simulink model "c_citation"  (R2020a)
settings: Solver=ode5  StartTime=0.0  StopTime=inf  FixedStep=0.01  RelTol=1e-3
InitFcn:
  | load('simulation_parameters');
values from neighbouring files (symbols this model uses):
  chord = 1.991    [citdata.mat]
  cv1 = 20000    [gear_params.m]
  cv2 = cv1    (= 20000)    [gear_params.m]
  cv3 = 4000    [gear_params.m]
  cv4 = 20000    [gear_params.m]
  deltagmax1 = 0.25    [gear_params.m]
  deltagmax2 = deltagmax1    (= 0.25)    [gear_params.m]
  deltagmax3 = 0.24    [gear_params.m]
  deltagmax4 = 0.02    [gear_params.m]
  ealphag = [0  0.2618  0.6981; 1  1.3  0.8]    [citdata.mat]
  ealphas = [0  0.2618  0.6981; 0.157  0.157  0.175]    [citdata.mat]
  g0 = 9.80665    [ac_genrl.mat]
  hDME = 0    [ac_genrl.mat]
  hGS = 0    [ac_genrl.mat]
  kt1 = 525020    [gear_params.m]
  kt2 = kt1    (= 525020)    [gear_params.m]
  kt3 = 457050    [gear_params.m]
  lh = 5.53    [citdata.mat]
  matbuaf = [0  -0.1745  0.4363; 0  -0.1  -0.1; 0.6981  -0.1  -0.1]    [citdata.mat]
  matdaf = [0 0 0.2618 0.6981 0.734842105263 0.771584210526 0.808326315789 0.845068421053 0.881810526316 0.918552631579 0.955294736842 0.992036842105 ... (529 elements, 23x23)]    [citdata.mat]
  matdam = [0 0.05 0.15 0.25 0.35 0.45 0.55 0.65 0.75 0.803571428571 0.857142857143 0.910714285714 ... (529 elements, 23x23)]    [citdata.mat]
  matdbbf = [0 0 0.6981 0.74464 0.79118 0.83772 0.88426 0.9308 0.97734 1.02388 1.07042 1.11696 ... (324 elements, 18x18)]    [citdata.mat]
  matdeaf = [0 0 0.2618 0.6981 0.734842105263 0.771584210526 0.808326315789 0.845068421053 0.881810526316 0.918552631579 0.955294736842 0.992036842105 ... (529 elements, 23x23)]    [citdata.mat]
  matdgaf = [0 0 0.2618 0.6981 -0.1745 -0.0175 -0.008 -0.009 0.4363 -0.0175 -0.008 -0.009 ... (16 elements, 4x4)]    [citdata.mat]
  matdqaf = [0 0 0.2618 0.6981 0.734842105263 0.771584210526 0.808326315789 0.845068421053 0.881810526316 0.918552631579 0.955294736842 0.992036842105 ... (529 elements, 23x23)]    [citdata.mat]
  matduaf = [0 0 0.2618 0.6981 0.734842105263 0.771584210526 0.808326315789 0.845068421053 0.881810526316 0.918552631579 0.955294736842 0.992036842105 ... (529 elements, 23x23)]    [citdata.mat]
  matdwaw = [0 0 0.1745 0.3491 0.5236 0.6458 1.2916 -0.1745 0 0.0018 0.0046 0.0088 ... (49 elements, 7x7)]    [citdata.mat]
  matedhr = [0 1 1 0.71 2 0.51 3 0.34 5 0.12 7.5 0.03 ... (20 elements, 2x10)]    [citdata.mat]
  mateif = [0  0.2618  0.6981; 0  -0.075  -0.075]    [citdata.mat]
  matelhr = [0 1 1 0.95 2 0.91 3 0.84 5 0.71 7.5 0.35 ... (20 elements, 2x10)]    [citdata.mat]
  matemhr = [0 1 1 0.9 2 0.8 3 0.7 5 0.5 7.5 0.25 ... (20 elements, 2x10)]    [citdata.mat]
  matemv1 = [0  90  100; 0  1  1]    [citdata.mat]
  matemv2 = [20  75  90; 0  1  1]    [citdata.mat]
  matemve = [0  90  100; 0  1  1]    [citdata.mat]
  matetam = [0  -0.1745  0.4363; 0  -0.04  -0.04; 1  -0.04  -0.04]    [citdata.mat]
  mateuaf = [0 0 0.6981 0.733005 0.76791 0.802815 0.83772 0.872625 0.90753 0.942435 0.97734 1.012245 ... (529 elements, 23x23)]    [citdata.mat]
  matfaaf = [0 0 0.2618 0.6981 0.734842105263 0.771584210526 0.808326315789 0.845068421053 0.881810526316 0.918552631579 0.955294736842 0.992036842105 ... (529 elements, 23x23)]    [citdata.mat]
  matfaxl = [0.15  0.35; 1  1]    [citdata.mat]
  matibaf = [0 0 0.2618 0.6981 -0.2 -0.119 -0.117 -0.108 0.3 -0.059 -0.052 -0.038 ... (16 elements, 4x4)]    [citdata.mat]
  matibb = [0 0 0.2618 1.571 3.142 -0.2 0 0 0.074 0.124 0 0 ... (50 elements, 5x10)]    [citdata.mat]
  matibmh = [0 0 15000 17142.8571429 19285.7142857 21428.5714286 23571.4285714 25714.2857143 27857.1428571 30000 0 0 ... (100 elements, 10x10)]    [citdata.mat]
  matipaf = [0  -0.1745  0.4363; 0  -0.44  -0.44; 0.6981  -0.44  -0.44]    [citdata.mat]
  matipmh = [0 0 15000 17142.8571429 19285.7142857 21428.5714286 23571.4285714 25714.2857143 27857.1428571 30000 0 0 ... (100 elements, 10x10)]    [citdata.mat]
  matiraf = [0 0 0.2618 0.6981 -0.2 0.05 -0.03 0.01 0.3 0.3 0.37 0.41 ... (16 elements, 4x4)]    [citdata.mat]
  matiuaf = [0  -0.2  0.3; 0  0.052  -0.003; 0.6981  0.052  -0.003]    [citdata.mat]
  matiwaf = [0  -0.1745  0.4363; 0  -0.185  -0.185; 0.6981  -0.185  -0.185]    [citdata.mat]
  matlaf = [0 0 0.2618 0.6981 0.734842105263 0.771584210526 0.808326315789 0.845068421053 0.881810526316 0.918552631579 0.955294736842 0.992036842105 ... (529 elements, 23x23)]    [citdata.mat]
  matlam = [0 0.05 0.15 0.25 0.35 0.45 0.55 0.65 0.75 0.803571428571 0.857142857143 0.910714285714 ... (529 elements, 23x23)]    [citdata.mat]
  matleaf = [0 0 0.2618 0.6981 0.734842105263 0.771584210526 0.808326315789 0.845068421053 0.881810526316 0.918552631579 0.955294736842 0.992036842105 ... (529 elements, 23x23)]    [citdata.mat]
  matleam = [0  -0.1745  0.4363; 0  0.58  0.58; 1  0.58  0.58]    [citdata.mat]
  matlgaf = [0 0 0.2618 0.6981 -0.1745 0.045 0.105 0.14 0.4363 0.045 0.105 0.14 ... (16 elements, 4x4)]    [citdata.mat]
  matlqaf = [0 0 0.2618 0.6981 0.734842105263 0.771584210526 0.808326315789 0.845068421053 0.881810526316 0.918552631579 0.955294736842 0.992036842105 ... (529 elements, 23x23)]    [citdata.mat]
  matluaf = [0 0 0.2618 0.6981 0.734842105263 0.771584210526 0.808326315789 0.845068421053 0.881810526316 0.918552631579 0.955294736842 0.992036842105 ... (529 elements, 23x23)]    [citdata.mat]
  matmaaf = [0 0 0.2618 0.6981 0.734842105263 0.771584210526 0.808326315789 0.845068421053 0.881810526316 0.918552631579 0.955294736842 0.992036842105 ... (484 elements, 22x22)]    [citdata.mat]
  matmaam = [0 0.05 0.15 0.25 0.35 0.45 0.55 0.65 0.75 0.803571428571 0.857142857143 0.910714285714 ... (484 elements, 22x22)]    [citdata.mat]
  matmaf = [0 0 0.2618 0.6981 0.734842105263 0.771584210526 0.808326315789 0.845068421053 0.881810526316 0.918552631579 0.955294736842 0.992036842105 ... (529 elements, 23x23)]    [citdata.mat]
  matmam = [0 0.05 0.15 0.25 0.35 0.45 0.55 0.65 0.75 0.803571428571 0.857142857143 0.910714285714 ... (529 elements, 23x23)]    [citdata.mat]
  matmbbf = [0 0 0.6981 0.74464 0.79118 0.83772 0.88426 0.9308 0.97734 1.02388 1.07042 1.11696 ... (324 elements, 18x18)]    [citdata.mat]
  matmeaf = [0 0 0.2618 0.6981 0.734842105263 0.771584210526 0.808326315789 0.845068421053 0.881810526316 0.918552631579 0.955294736842 0.992036842105 ... (529 elements, 23x23)]    [citdata.mat]
  matmeam = [0 0 1 1.05 1.1 1.15 1.2 1.25 1.3 1.35 1.4 1.45 ... (529 elements, 23x23)]    [citdata.mat]
  matmgaf = [0 0 0.2618 0.6981 -0.1745 -0.01 -0.024 -0.035 0.4363 -0.01 -0.024 -0.035 ... (16 elements, 4x4)]    [citdata.mat]
  matmqaf = [0 0 0.2618 0.6981 0.734842105263 0.771584210526 0.808326315789 0.845068421053 0.881810526316 0.918552631579 0.955294736842 0.992036842105 ... (529 elements, 23x23)]    [citdata.mat]
  matmrbr = [0  0  0.5236; 0  0  0; 0.384  0.001  0.001]    [citdata.mat]
  matnbab = [0 0 0.2618 1.571 3.142 -0.2 0 0 -0.0199 -0.1049 0 0 ... (25 elements, 5x5)]    [citdata.mat]
  matnbaf = [0  -0.2  0.3; 0  0.105  0.18; 0.6981  0.105  0.18]    [citdata.mat]
  matnbmh = [0 0 15000 17142.8571429 19285.7142857 21428.5714286 23571.4285714 25714.2857143 27857.1428571 30000 0 0 ... (100 elements, 10x10)]    [citdata.mat]
  matnpaf = [0 0 0.2618 0.6981 -0.2 0.03 0.03 0.05 0.3 -0.12 -0.12 -0.2 ... (16 elements, 4x4)]    [citdata.mat]
  matnpmh = [0 0 15000 17142.8571429 19285.7142857 21428.5714286 23571.4285714 25714.2857143 27857.1428571 30000 0 0 ... (100 elements, 10x10)]    [citdata.mat]
  matnraf = [0  -0.1745  0.4363; 0  -0.21  -0.21; 0.6981  -0.21  -0.21]    [citdata.mat]
  matnuaf = [0  -0.1745  0.4363; 0  -0.101  -0.101; 0.6981  -0.101  -0.101]    [citdata.mat]
  matnwaf = [0 0 0.2618 0.6981 -0.2 -0.02 -0.037 -0.049 0.3 0.03 0.043 0.036 ... (16 elements, 4x4)]    [citdata.mat]
  matnwmh = [0 0 15000 17142.8571429 19285.7142857 21428.5714286 23571.4285714 25714.2857143 27857.1428571 30000 0 0 ... (100 elements, 10x10)]    [citdata.mat]
  matqlaf = [0  -0.1745  0.4363; 0  -1  -1; 0.6981  -1  -1]    [citdata.mat]
  matquaf = [0 0 0.6981 0.733005 0.76791 0.802815 0.83772 0.872625 0.90753 0.942435 0.97734 1.012245 ... (529 elements, 23x23)]    [citdata.mat]
  matqxl = [0.15  0.35; 1  1]    [citdata.mat]
  matqxm = [0.15  0.35; 1  1]    [citdata.mat]
  matrtam = [0  -0.1745  0.4363; 0  0.011  0.011; 1  0.011  0.011]    [citdata.mat]
  matruaf = [0  -0.1745  0.4363; 0  0.2  0.2; 0.6981  0.2  0.2]    [citdata.mat]
  matrumh = [0 0 15000 17142.8571429 19285.7142857 21428.5714286 23571.4285714 25714.2857143 27857.1428571 30000 0 0 ... (100 elements, 10x10)]    [citdata.mat]
  matuut = [0  0.5  1; 0  1.35  1]    [citdata.mat]
  matwtam = [0  -0.1745  0.4363; 0  0.011  0.011; 1  0.011  0.011]    [citdata.mat]
  matybab = [0 0 0.2618 1.571 3.142 -0.2 0 0 0.34 0.75 0 0 ... (25 elements, 5x5)]    [citdata.mat]
  matybaf = [0  -0.1745  0.4363; 0  -0.75  -0.75; 0.6981  -0.75  -0.75]    [citdata.mat]
  matyraf = [0  -0.1745  0.4363; 0  0.85  0.85; 0.6981  0.85  0.85]    [citdata.mat]
  matyuaf = [0  -0.1745  0.4363; 0  0.23  0.23; 0.6981  0.23  0.23]    [citdata.mat]
  matywaf = [0  -0.1745  0.4363; 0  -0.04  -0.04; 0.6981  -0.04  -0.04]    [citdata.mat]
  murol = 0.03*10    (= 0.3)    [gear_params.m]
  P1 = 2000    [gear_params.m]
  P2 = P1    (= 2000)    [gear_params.m]
  P3 = 2550    [gear_params.m]
  P4 = 40000    [gear_params.m]
  psiLOC = 0    [ac_genrl.mat]
  pstat0 = 101325    [ac_genrl.mat]
  S = 24.99    [citdata.mat]
  span = 13.325    [citdata.mat]
  T0 = 288.15    [ac_genrl.mat]
  tilteng = [0 0]    [citdata.mat]
  toweng = [0 0]    [citdata.mat]
  vdommyr37 = [0  0.2618  0.6981; 0  0.025  0]    [citdata.mat]
  vdommyr38 = [0  0.2618  0.6981; -0.01  0  -0.01]    [citdata.mat]
  Vw915 = 0    [initcit.m]
  winddir = 45*(pi/180)    (= 0.785398163397)    [initcit.m]
  xcgref = 6.5    [citdata.mat]
  xDME = 0    [ac_genrl.mat]
  xeng = [8.407 8.407]    [citdata.mat]
  xGS = 0    [ac_genrl.mat]
  xiacc = 3.2    [ac_genrl.mat]
  xl1 = xcg-6.858    [gear_params.m]
  xl2 = xcg-6.858    [gear_params.m]
  xl3 = xcg-2.0752    [gear_params.m]
  xl4 = xcg-12.742    [gear_params.m]
  xLOC = 0    [ac_genrl.mat]
  ycgref = 0    [citdata.mat]
  yDME = 0    [ac_genrl.mat]
  yeng = [3 -3]    [citdata.mat]
  yGS = 0    [ac_genrl.mat]
  yiacc = 0    [ac_genrl.mat]
  yl1 = 1.918    [gear_params.m]
  yl2 = -1.918    [gear_params.m]
  yl3 = 0    [gear_params.m]
  ... (+9 more)
undefined symbols (not defined in the file or in its folder): Deng, massinit, matff, matn1d, matn2d, matthr, u0, ut0, x0, xt0
(part 2 of 5)

== system c_citation/Cessna Citation 500/Citation model DASMAT/AIRCRAFT MODEL/AFM/FMaerodims ==
  Ca : Inport
  Cadot : Inport  Port=2
  Cbdot : Inport  Port=3
  x : Inport  Port=4
  yad1 : Inport  Port=5
  Prod : Product  InputSameDT=on  SaturateOnIntegerOverflow=on  OutDataTypeStr=Inherit: Same as first input
  Prod1 : Product  Inputs=3  InputSameDT=on  SaturateOnIntegerOverflow=on  OutDataTypeStr=Inherit: Same as first input
  Prod2 : Product  Inputs=3  InputSameDT=on  SaturateOnIntegerOverflow=on  OutDataTypeStr=Inherit: Same as first input
  b/V : Fcn  Expr=span/u[4]
  c/V : Fcn  Expr=chord/u[4]
  dims : Subsystem
  dims1 : Subsystem
  dims2 : Subsystem
  qdyn*S : Fcn  Expr=u[2]*S
  FMa : Outport  VectorParamsAs1DForOutWhenUnconnected=off
  FMadot : Outport  Port=2  VectorParamsAs1DForOutWhenUnconnected=off
  FMbdot : Outport  Port=3  VectorParamsAs1DForOutWhenUnconnected=off
  wires:
  Ca/1 -> Prod/1
  Prod/1 -> dims/1(FM/length)
  dims/1(FM) -> FMa/1
  yad1/1 -> qdyn*S/1
  Cbdot/1 -> Prod2/1
  qdyn*S/1 -> Prod2/2, Prod1/2, Prod/2
  Cadot/1 -> Prod1/1
  Prod1/1 -> dims1/1(F FM/length)
  dims1/1(FM) -> FMadot/1
  Prod2/1 -> dims2/1(F FM/length)
  dims2/1(FM) -> FMbdot/1
  x/1 -> b/V/1, c/V/1
  c/V/1 -> Prod1/3
  b/V/1 -> Prod2/3

== system c_citation/Cessna Citation 500/Citation model DASMAT/AIRCRAFT MODEL/AFM/FMgustdims ==
  Cag : Inport
  yad1 : Inport  Port=2
  Prod : Product  InputSameDT=on  SaturateOnIntegerOverflow=on  OutDataTypeStr=Inherit: Same as first input
  dims : Subsystem
  qdyn*S : Fcn  Expr=u[2]*S
  FMag : Outport  VectorParamsAs1DForOutWhenUnconnected=off
  wires:
  Cag/1 -> Prod/1
  Prod/1 -> dims/1(F M/length)
  yad1/1 -> qdyn*S/1
  dims/1(FM) -> FMag/1
  qdyn*S/1 -> Prod/2

== system c_citation/Cessna Citation 500/Citation model DASMAT/AIRCRAFT MODEL/AFM/Gust axes-cg transformation ==
  Cag model : Inport
  "x " : Inport  Port=2
  massinit : Inport  Port=3
  Demux1 : Demux  Outputs=[3 3 3 3]
      settings: DisplayOption=none
  Fag transformation : S-Function  FunctionName=ac_axes  Parameters=axes_CFMgust  SFunctionDeploymentMode=off  EnableBusSupport=off
  Mag transformation : S-Function  FunctionName=ac_axes  Parameters=axes_CFMgust  SFunctionDeploymentMode=off  EnableBusSupport=off
  Mux1 : Mux  Inputs=[12 3]
  Mux2 : Mux  Inputs=[12 3]
  Mux3 : Mux  Inputs=[3 3]
  Mux4 : Mux  Inputs=[12 1 1 1]
  Mux5 : Mux  Inputs=[12 12]
  Mux6 : Mux  Inputs=3
  Sum : Sum  Inputs=+-  InputSameDT=on  SaturateOnIntegerOverflow=on  OutDataTypeStr=Inherit: Same as first input
  Sum1 : Sum  InputSameDT=on  SaturateOnIntegerOverflow=on  OutDataTypeStr=Inherit: Same as first input
  Terminator_{1..5} (5 alike) : Terminator
  delta CLLbody : Fcn  Expr=(u[2]*u[6]-u[3]*u[5])/span
  delta CMbody : Fcn  Expr=(-u[1]*u[6]+u[3]*u[4])/chord
  delta CNbody : Fcn  Expr=(u[1]*u[5]-u[2]*u[4])/span
  delta Mag transformation : S-Function  FunctionName=ac_axes  Parameters=2  SFunctionDeploymentMode=off  EnableBusSupport=off
  gust : Demux  Outputs=[3 3]
      settings: DisplayOption=none
  mass cg inertia : Demux  Outputs=[1 3 4]
      settings: DisplayOption=none
  xref : Constant  Value=xcgref
  yref : Constant  Value=ycgref
  zref : Constant  Value=zcgref
  Cag : Outport  VectorParamsAs1DForOutWhenUnconnected=off
  wires:
  mass cg inertia/3 -> Terminator_5/1
  mass cg inertia/1 -> Terminator_4/1
  Demux1/4 -> Terminator_3/1
  Demux1/2 -> Terminator_2/1
  Demux1/1 -> Terminator_1/1
  Cag model/1 -> gust/1
  massinit/1 -> mass cg inertia/1
  gust/1 -> Mux1/2
  xref/1 -> Mux6/1
  yref/1 -> Mux6/2
  zref/1 -> Mux6/3
  mass cg inertia/2 -> Sum/2
  Mux6/1 -> Sum/1
  Fag transformation/1 -> Demux1/1, Mux5/1
  Mag transformation/1 -> Sum1/1
  Sum1/1 -> Mux5/2
  Mux5/1 -> Cag/1
  Mux1/1 -> Fag transformation/1
  delta Mag transformation/1 -> Sum1/2
  Mux2/1 -> Mag transformation/1
  Sum/1 -> Mux3/2
  gust/2 -> Mux2/2
  "x "/1 -> Mux2/1, Mux1/1, Mux4/1
  Mux3/1 -> delta CLLbody/1, delta CNbody/1, delta CMbody/1
  delta CLLbody/1 -> Mux4/2
  delta CMbody/1 -> Mux4/3
  delta CNbody/1 -> Mux4/4
  Demux1/3 -> Mux3/1
  Mux4/1 -> delta Mag transformation/1

== system c_citation/Cessna Citation 500/Citation model DASMAT/AIRCRAFT MODEL/EFM/Engine axes-cg transformation ==
  FMt model : Inport
  "x " : Inport  Port=2
  massinit : Inport  Port=3
  Demux : Demux  Outputs=[3 3 3 3]
      settings: DisplayOption=none
  Ft transformation : S-Function  FunctionName=ac_axes  Parameters=2  SFunctionDeploymentMode=off  EnableBusSupport=off
  Mt transformation : S-Function  FunctionName=ac_axes  Parameters=2  SFunctionDeploymentMode=off  EnableBusSupport=off
  Mux1 : Mux  Inputs=[12 3]
  Mux2 : Mux  Inputs=[12 3]
  Mux3 : Mux  Inputs=[3 3]
  Mux4 : Mux  Inputs=[12 1 1 1]
  Mux5 : Mux  Inputs=[12 12]
  "Neg " : Gain  Gain=-1  SaturateOnIntegerOverflow=on  OutDataTypeStr=Inherit: Same as input  ParamDataTypeStr=Inherit: Same as input
  Sum1 : Sum  InputSameDT=on  SaturateOnIntegerOverflow=on  OutDataTypeStr=Inherit: Same as first input
  Terminator_{1..5} (5 alike) : Terminator
  delta LLbody : Fcn  Expr=u[2]*u[6]-u[3]*u[5]
  delta Mbody : Fcn  Expr=-u[1]*u[6]+u[3]*u[4]
  delta Mt transformation : S-Function  FunctionName=ac_axes  Parameters=2  SFunctionDeploymentMode=off  EnableBusSupport=off
  delta Nbody : Fcn  Expr=u[1]*u[5]-u[2]*u[4]
  engine : Demux  Outputs=[3 3]
      settings: DisplayOption=none
  mass cg inertia : Demux  Outputs=[1 3 4]
      settings: DisplayOption=none
  FMt : Outport  VectorParamsAs1DForOutWhenUnconnected=off
  wires:
  mass cg inertia/3 -> Terminator_5/1
  mass cg inertia/1 -> Terminator_4/1
  Demux/4 -> Terminator_3/1
  Demux/2 -> Terminator_2/1
  Demux/1 -> Terminator_1/1
  FMt model/1 -> engine/1
  massinit/1 -> mass cg inertia/1
  engine/1 -> Mux1/2
  Ft transformation/1 -> Demux/1, Mux5/1
  Mt transformation/1 -> Sum1/1
  Sum1/1 -> Mux5/2
  Mux5/1 -> FMt/1
  Mux1/1 -> Ft transformation/1
  delta Mt transformation/1 -> Sum1/2
  Mux2/1 -> Mt transformation/1
  engine/2 -> Mux2/2
  "x "/1 -> Mux2/1, Mux1/1, Mux4/1
  Mux3/1 -> delta LLbody/1, delta Nbody/1, delta Mbody/1
  delta LLbody/1 -> Mux4/2
  delta Mbody/1 -> Mux4/3
  delta Nbody/1 -> Mux4/4
  Mux4/1 -> delta Mt transformation/1
  Demux/3 -> Mux3/1
  mass cg inertia/2 -> "Neg "/1
  "Neg "/1 -> Mux3/2

== system c_citation/Cessna Citation 500/Citation model DASMAT/AIRCRAFT MODEL/EFM/Engmod ==
  x : Inport
  ut : Inport  Port=2
  yatm : Inport  Port=3
  yad1 : Inport  Port=4
  yad2 : Inport  Port=5
  Citation eng_mod : Subsystem
  Mux : Mux  Inputs=[12 2 8 2 8]
  FMt : Outport  VectorParamsAs1DForOutWhenUnconnected=off
  ypp : Outport  Port=2  VectorParamsAs1DForOutWhenUnconnected=off
  wires:
  x/1 -> Mux/1
  ut/1 -> Mux/2
  yatm/1 -> Mux/3
  yad1/1 -> Mux/4
  yad2/1 -> Mux/5
  Mux/1 -> Citation eng_mod/1(In1)
  Citation eng_mod/1(Out1) -> FMt/1
  Citation eng_mod/2(ypp) -> ypp/1

== system c_citation/Cessna Citation 500/Citation model DASMAT/AIRCRAFT MODEL/EQM/CFMa correction ==
  xdot : Inport
  FMa : Inport  Port=2
  FMadot : Inport  Port=3
  FMbdot : Inport  Port=4
  Prod2 : Product  InputSameDT=on  SaturateOnIntegerOverflow=on  OutDataTypeStr=Inherit: Same as first input
  Prod3 : Product  InputSameDT=on  SaturateOnIntegerOverflow=on  OutDataTypeStr=Inherit: Same as first input
  Sum1 : Sum  Inputs=+++  InputSameDT=on  SaturateOnIntegerOverflow=on  OutDataTypeStr=Inherit: Same as first input
  Terminator_{1..10} (10 alike) : Terminator
  derivatives : Demux  Outputs=12
      settings: DisplayOption=none
  FMa corrected : Outport  VectorParamsAs1DForOutWhenUnconnected=off
  wires:
  derivatives/12 -> Terminator_10/1
  derivatives/11 -> Terminator_9/1
  derivatives/10 -> Terminator_8/1
  derivatives/9 -> Terminator_7/1
  derivatives/8 -> Terminator_6/1
  derivatives/7 -> Terminator_5/1
  derivatives/4 -> Terminator_4/1
  derivatives/3 -> Terminator_3/1
  derivatives/2 -> Terminator_2/1
  derivatives/1 -> Terminator_1/1
  xdot/1 -> derivatives/1
  Sum1/1 -> FMa corrected/1
  FMa/1 -> Sum1/1
  FMbdot/1 -> Prod3/1
  FMadot/1 -> Prod2/1
  Prod2/1 -> Sum1/2
  Prod3/1 -> Sum1/3
  derivatives/5 -> Prod2/2
  derivatives/6 -> Prod3/2

== system c_citation/Cessna Citation 500/Citation model DASMAT/AIRCRAFT MODEL/EQM/State Derivatives ==
  note: mass
  note: inertia
  x : Inport
  FMtot : Inport  Port=2
  FMadot : Inport  Port=3
  FMbdot : Inport  Port=4
  massinit : Inport  Port=5
  wind : Inport  Port=6
  Mux1 : Mux  Inputs=[12 12]
  Mux2 : Mux  Inputs=[3 3 3 3]
  Terminator_1 : Terminator
  Vabdot : Subsystem
  aero1 : Demux  Outputs=[12 12]
      settings: DisplayOption=none
  aero2 : Demux  Outputs=[12 12]
      settings: DisplayOption=none
  eulerdot : Subsystem
  hxydot : Subsystem
  mass properties : Subsystem
  pqrdot : Subsystem
  states transformation : Subsystem
  total : Demux  Outputs=[12 12]
      settings: DisplayOption=none
  xdot : Outport  VectorParamsAs1DForOutWhenUnconnected=off
  yuvw : Outport  Port=2  VectorParamsAs1DForOutWhenUnconnected=off
  FMtot corrected : Outport  Port=3  VectorParamsAs1DForOutWhenUnconnected=off
  wires:
  states transformation/3(ydl) -> Terminator_1/1
  wind/1 -> hxydot/2(wind), Vabdot/7(wind)
  total/1 -> Vabdot/3(Ftot)
  states transformation/2(yuvw) -> hxydot/1(yuvw), yuvw/1
  Mux1/1 -> FMtot corrected/1
  hxydot/1(hxydot) -> Mux2/4
  eulerdot/1(eulerdot) -> Mux2/3
  pqrdot/2(Mtot corrected) -> Mux1/2
  pqrdot/1(pqrdot) -> Mux2/1
  Vabdot/2(Ftot corrected) -> Mux1/1
  aero2/1 -> Vabdot/5(Fbdot)
  total/2 -> pqrdot/2(Mtot)
  mass properties/2(inertia) -> pqrdot/5(inertia)
  mass properties/1(mass) -> Vabdot/6(mass)
  aero1/1 -> Vabdot/4(Fadot)
  states transformation/1(ypqr) -> pqrdot/1(ypqr), Vabdot/2(ypqr)
  x/1 -> Vabdot/1(x), eulerdot/1(x), states transformation/1(x)
  aero2/2 -> pqrdot/4(Mbdot)
  aero1/2 -> pqrdot/3(Madot)
  Vabdot/1(Vabdot) -> pqrdot/6(Vabdot), Mux2/2
  FMbdot/1 -> aero2/1
  FMadot/1 -> aero1/1
  FMtot/1 -> total/1
  massinit/1 -> mass properties/1(massinit)
  Mux2/1 -> xdot/1

== system c_citation/Cessna Citation 500/Citation model DASMAT/AIRCRAFT MODEL/LANDING GEAR/Gear axes-cg transformation ==
  FMt model : Inport
  "x " : Inport  Port=2
  massinit : Inport  Port=3
  Demux : Demux  Outputs=[3 3 3 3]
      settings: DisplayOption=none
  Ft transformation : S-Function  FunctionName=ac_axes  Parameters=2  SFunctionDeploymentMode=off  EnableBusSupport=off
  Gear Forces and Moments : Demux  Outputs=[3 3]
      settings: DisplayOption=none
  Mt transformation : S-Function  FunctionName=ac_axes  Parameters=2  SFunctionDeploymentMode=off  EnableBusSupport=off
  Mux1 : Mux  Inputs=[12 3]
  Mux2 : Mux  Inputs=[12 3]
  Mux3 : Mux  Inputs=[3 3]
  Mux4 : Mux  Inputs=[12 1 1 1]
  Mux5 : Mux  Inputs=[12 12]
  "Neg " : Gain  Gain=-1  SaturateOnIntegerOverflow=on  OutDataTypeStr=Inherit: Same as input  ParamDataTypeStr=Inherit: Same as input
  Scope3 : Scope
  Scope4 : Scope
  Terminator_{1..6} (6 alike) : Terminator
  delta LLbody : Fcn  Expr=u[2]*u[6]-u[3]*u[5]
  delta Mbody : Fcn  Expr=-u[1]*u[6]+u[3]*u[4]
  delta Mt transformation : S-Function  FunctionName=ac_axes  Parameters=2  SFunctionDeploymentMode=off  EnableBusSupport=off
  delta Nbody : Fcn  Expr=u[1]*u[5]-u[2]*u[4]
  mass cg inertia : Demux  Outputs=[1 3 4]
      settings: DisplayOption=none
  FMt : Outport  VectorParamsAs1DForOutWhenUnconnected=off
  wires:
  mass cg inertia/3 -> Terminator_5/1
  mass cg inertia/1 -> Terminator_4/1
  Demux/4 -> Terminator_3/1
  Demux/2 -> Terminator_2/1
  Demux/1 -> Terminator_1/1
  FMt model/1 -> Gear Forces and Moments/1
  massinit/1 -> mass cg inertia/1
  Gear Forces and Moments/1 -> Mux1/2
  Ft transformation/1 -> Demux/1, Mux5/1
  Mux5/1 -> FMt/1
  Mux1/1 -> Ft transformation/1
  Mux2/1 -> Mt transformation/1
  Gear Forces and Moments/2 -> Mux2/2
  "x "/1 -> Mux2/1, Mux1/1, Mux4/1
  Mux3/1 -> delta LLbody/1, delta Nbody/1, delta Mbody/1
  delta LLbody/1 -> Mux4/2
  delta Mbody/1 -> Mux4/3
  delta Nbody/1 -> Mux4/4
  Mux4/1 -> delta Mt transformation/1
  Demux/3 -> Mux3/1
  mass cg inertia/2 -> "Neg "/1
  "Neg "/1 -> Mux3/2
  Mt transformation/1 -> Scope3/1, Mux5/2, Scope4/1
  delta Mt transformation/1 -> Terminator_6/1

== system c_citation/Cessna Citation 500/Citation model DASMAT/AIRCRAFT MODEL/LANDING GEAR/Landing Gear model ==
  note: NLR Model
  x : Inport
  xdot : Inport  Port=2
  terrain elevation : Inport  Port=3
  Correct for terrain elevation : Subsystem
  Left Main Gear : Subsystem
  Mux : Mux  Inputs=2
  Mux1 : Mux  Inputs=2
  Nose Gear : Subsystem
  Right Main Gear : Subsystem
  Sum : Sum  Inputs=++++  InputSameDT=on  SaturateOnIntegerOverflow=on  OutDataTypeStr=Inherit: Same as first input
  Sum1 : Sum  Inputs=++++  InputSameDT=on  SaturateOnIntegerOverflow=on  OutDataTypeStr=Inherit: Same as first input
  Tail Scraper : Subsystem
  hdot selector : Selector  IndexOptions=Index vector (dialog)  Indices=[10]  OutputSizes=1
  Forces and Moments : Outport  VectorParamsAs1DForOutWhenUnconnected=off
  wires:
  xdot/1 -> hdot selector/1
  Mux/1 -> Left Main Gear/1(Inputs), Nose Gear/1(Inputs), Right Main Gear/1(Inputs), Tail Scraper/1(Inputs)
  Mux1/1 -> Forces and Moments/1
  Correct for terrain elevation/1(x corrected) -> Mux/1
  x/1 -> Correct for terrain elevation/1(x)
  Tail Scraper/1(FX FY FZ) -> Sum/4
  Tail Scraper/2(L M N) -> Sum1/4
  Right Main Gear/1(FX FY FZ) -> Sum/3
  Nose Gear/2(L M N) -> Sum1/2
  Sum1/1 -> Mux1/2
  Sum/1 -> Mux1/1
  Left Main Gear/1(FX FY FZ) -> Sum/1
  Left Main Gear/2(L M N) -> Sum1/1
  Nose Gear/1(FX FY FZ) -> Sum/2
  Right Main Gear/2(L M N) -> Sum1/3
  terrain elevation/1 -> Correct for terrain elevation/2(terr elev)
  hdot selector/1 -> Mux/2

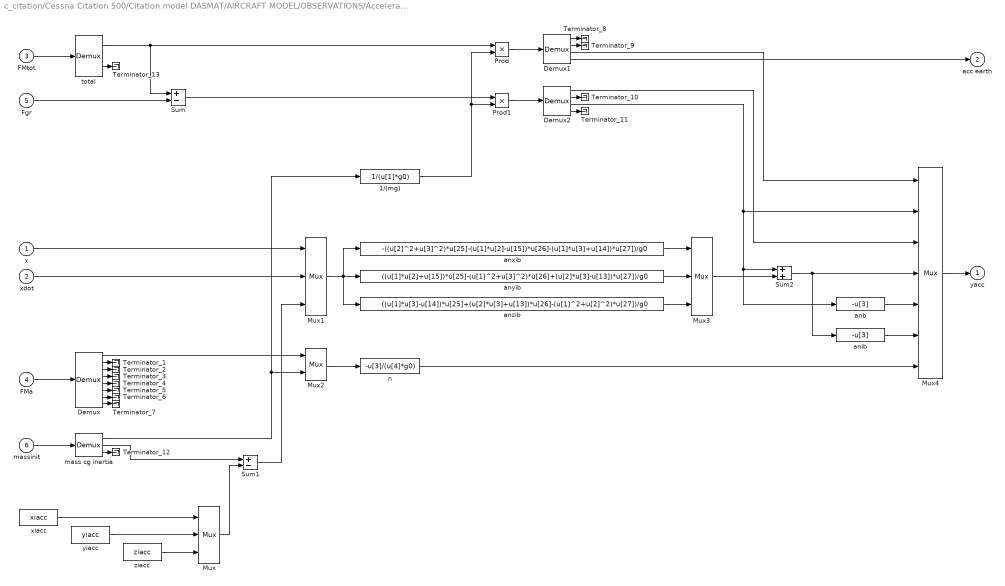
== system c_citation/Cessna Citation 500/Citation model DASMAT/AIRCRAFT MODEL/OBSERVATIONS/Acceleration ==
  x : Inport
  xdot : Inport  Port=2
  FMtot : Inport  Port=3
  FMa : Inport  Port=4
  Fgr : Inport  Port=5
  massinit : Inport  Port=6
  1/(mg) : Fcn  Expr=1/(u[1]*g0)
  Demux : Demux  Outputs=[3 3 3 3 3 3 3 3]
      settings: DisplayOption=none
  Demux1 : Demux  Outputs=[3 3 3 3]
      settings: DisplayOption=none
  Demux2 : Demux  Outputs=[3 3 3 3]
      settings: DisplayOption=none
  Mux : Mux  Inputs=3
  Mux1 : Mux  Inputs=[12 12 3]
  Mux2 : Mux  Inputs=[3 1]
  Mux3 : Mux  Inputs=3
  Mux4 : Mux  Inputs=[3 3 3 3 1 1 1]
  Prod : Product  InputSameDT=on  SaturateOnIntegerOverflow=on  OutDataTypeStr=Inherit: Same as first input
  Prod1 : Product  InputSameDT=on  SaturateOnIntegerOverflow=on  OutDataTypeStr=Inherit: Same as first input
  Sum : Sum  Inputs=+-  InputSameDT=on  SaturateOnIntegerOverflow=on  OutDataTypeStr=Inherit: Same as first input
  Sum1 : Sum  Inputs=+-  InputSameDT=on  SaturateOnIntegerOverflow=on  OutDataTypeStr=Inherit: Same as first input
  Sum2 : Sum  InputSameDT=on  SaturateOnIntegerOverflow=on  OutDataTypeStr=Inherit: Same as first input
  Terminator_{1..13} (13 alike) : Terminator
  anb : Fcn  Expr=-u[3]
  anib : Fcn  Expr=-u[3]
  anxib : Fcn  Expr=-((u[2]^2+u[3]^2)*u[25]-(u[1]*u[2]-u[15])*u[26]-(u[1]*u[3]+u[14])*u[27])/g0
  anyib : Fcn  Expr=((u[1]*u[2]+u[15])*u[25]-(u[1]^2+u[3]^2)*u[26]+(u[2]*u[3]-u[13])*u[27])/g0
  anzib : Fcn  Expr=((u[1]*u[3]-u[14])*u[25]+(u[2]*u[3]+u[13])*u[26]-(u[1]^2+u[2]^2)*u[27])/g0
  mass cg inertia : Demux  Outputs=[1 3 4]
      settings: DisplayOption=none
  n : Fcn  Expr=-u[3]/(u[4]*g0)
  total : Demux  Outputs=[12 12]
      settings: DisplayOption=none
  xiacc : Constant  Value=xiacc
  yiacc : Constant  Value=yiacc
  ziacc : Constant  Value=ziacc
  yacc : Outport  VectorParamsAs1DForOutWhenUnconnected=off
  acc earth : Outport  Port=2  VectorParamsAs1DForOutWhenUnconnected=off
  wires:
  total/2 -> Terminator_13/1
  mass cg inertia/3 -> Terminator_12/1
  Demux2/4 -> Terminator_11/1
  Demux2/2 -> Terminator_10/1
  Demux1/2 -> Terminator_9/1
  Demux1/1 -> Terminator_8/1
  Demux/8 -> Terminator_7/1
  Demux/7 -> Terminator_6/1
  Demux/6 -> Terminator_5/1
  Demux/5 -> Terminator_4/1
  Demux/4 -> Terminator_3/1
  Demux/3 -> Terminator_2/1
  Demux/2 -> Terminator_1/1
  Mux4/1 -> yacc/1
  anb/1 -> Mux4/5
  Sum1/1 -> Mux1/3
  x/1 -> Mux1/1
  xdot/1 -> Mux1/2
  mass cg inertia/2 -> Sum1/1
  anzib/1 -> Mux3/3
  anxib/1 -> Mux3/1
  anyib/1 -> Mux3/2
  Mux2/1 -> n/1
  massinit/1 -> mass cg inertia/1
  xiacc/1 -> Mux/1
  yiacc/1 -> Mux/2
  ziacc/1 -> Mux/3
  1/(mg)/1 -> Prod1/2, Prod/2
  Sum/1 -> Prod1/1
  Mux1/1 -> anxib/1, anzib/1, anyib/1
  mass cg inertia/1 -> Mux2/2, 1/(mg)/1
  Mux/1 -> Sum1/2
  Mux3/1 -> Sum2/2
  Sum2/1 -> anib/1, Mux4/4
  FMa/1 -> Demux/1
  Fgr/1 -> Sum/2
  anib/1 -> Mux4/6
  n/1 -> Mux4/7
  total/1 -> Sum/1, Prod/1
  FMtot/1 -> total/1
  Demux/1 -> Mux2/1
  Demux2/3 -> Mux4/2, Sum2/1, anb/1
  Demux1/3 -> Mux4/1
  Prod/1 -> Demux1/1
  Demux2/1 -> Mux4/3
  Prod1/1 -> Demux2/1
  Demux1/4 -> acc earth/1

== system c_citation/Cessna Citation 500/Citation model DASMAT/AIRCRAFT MODEL/OBSERVATIONS/Energy ==
  x : Inport
  xdot : Inport  Port=2
  yatm : Inport  Port=3
  Mux : Mux  Inputs=[12 12 8]
  Mux1 : Mux  Inputs=2
  spec energy : Fcn  Expr=u[10]+(u[4]*u[4])/(2*u[28])
  spec power : Fcn  Expr=u[22]+(u[4]*u[16])/u[28]
  ys : Outport  VectorParamsAs1DForOutWhenUnconnected=off
  wires:
  spec power/1 -> Mux1/2
  spec energy/1 -> Mux1/1
  x/1 -> Mux/1
  xdot/1 -> Mux/2
  Mux1/1 -> ys/1
  yatm/1 -> Mux/3
  Mux/1 -> spec power/1, spec energy/1

== system c_citation/Cessna Citation 500/Citation model DASMAT/AIRCRAFT MODEL/OBSERVATIONS/Flight-Path ==
  x : Inport
  xdot : Inport  Port=2
  yuvw : Inport  Port=3
  acc earth : Inport  Port=4
  Demux : Demux  Outputs=[3 3 3 3]
      settings: DisplayOption=none
  Mux : Mux  Inputs=[12 12 3 3]
  Mux1 : Mux  Inputs=[30 1 1]
  Mux2 : Mux  Inputs=17
  Terminator11 : Terminator
  Terminator12 : Terminator
  Terminator13 : Terminator
  Vground : Fcn  Expr=sqrt(u[23]*u[23]+u[24]*u[24]+u[22]*u[22])
  bank angle : Fcn  Expr=asin(sin(u[7])*cos(u[8]))
  chi : Fcn  Expr=atan2(u[26],u[25])
  chidot : Fcn  Expr=(u[25]*u[29]*g0-u[28]*g0*u[26])/(u[4]*u[4]-u[27]*u[27])
  chimagn : Fcn  Expr=0
  chitrue : Fcn  Expr=atan2(u[24],u[23])
  chitruedot : Fcn  Expr=(u[23]*u[29]*g0-u[28]*g0*u[24])/(u[31]*u[31]-u[22]*u[22])
  flightpath acc : Fcn  Expr=u[16]/g0
  gamma : Fcn  Expr=asin(-u[27]/u[4])
  gammadot : Fcn  Expr=(-u[4]*u[30]*g0+u[16]*u[27])/(u[4]*sqrt(u[4]*u[4]-u[27]*u[27]))
  gammatrue : Fcn  Expr=asin(u[22]/u[31])
  gammatruedot : Fcn  Expr=(u[31]*u[32]*g0-u[16]*u[22])/(u[31]*sqrt(u[31]*u[31]-u[22]*u[22]))
  gsdev : Fcn  Expr=atan2(u[10]-hGS,sqrt((xGS-u[11])*(xGS-u[11])+(yGS-u[12])*(yGS-u[12]))) - 3*pi/180
  locdev : Fcn  Expr=psiLOC - atan2(yLOC-u[12],xLOC-u[11])
  psimagn : Fcn  Expr=0
  range : Fcn  Expr=sqrt((u[11]-xDME)*(u[11]-xDME)+(u[12]-yDME)*(u[12]-yDME)+(u[10]-hDME)*(u[10]-hDME))
  vertical acc : Fcn  Expr=-u[30]
  yfp : Outport  VectorParamsAs1DForOutWhenUnconnected=off
  wires:
  Demux/3 -> Terminator13/1
  Demux/2 -> Terminator12/1
  Demux/1 -> Terminator11/1
  vertical acc/1 -> Mux1/3, Mux2/16
  Mux1/1 -> gammatruedot/1, chitruedot/1, gammatrue/1, chitrue/1
  Vground/1 -> Mux1/2, Mux2/15
  xdot/1 -> Mux/2
  Demux/4 -> Mux/3
  acc earth/1 -> Mux/4
  yuvw/1 -> Demux/1
  chi/1 -> Mux2/2
  Mux2/1 -> yfp/1
  gamma/1 -> Mux2/1
  gammadot/1 -> Mux2/3
  chidot/1 -> Mux2/4
  gammatrue/1 -> Mux2/5
  chitrue/1 -> Mux2/6
  gammatruedot/1 -> Mux2/7
  flightpath acc/1 -> Mux2/17
  range/1 -> Mux2/14
  locdev/1 -> Mux2/13
  gsdev/1 -> Mux2/12
  bank angle/1 -> Mux2/11
  psimagn/1 -> Mux2/10
  chimagn/1 -> Mux2/9
  chitruedot/1 -> Mux2/8
  x/1 -> Mux/1
  Mux/1 -> Mux1/1, gammadot/1, chi/1, gamma/1, chidot/1, gsdev/1, locdev/1, range/1, Vground/1, vertical acc/1, flightpath acc/1, bank angle/1, psimagn/1, chimagn/1

== system c_citation/Cessna Citation 500/Citation model DASMAT/AIRCRAFT MODEL/WIND//TURBULENCE/Logarithmic Wind model ==
  In1 : Inport
  He Selector : Selector  InputPortWidth=12  IndexOptions=Index vector (dialog)  Indices=[10]  OutputSizes=1
  Logarithmic Wind model : Subsystem
  Mux : Mux  Inputs=3
  Out1 : Outport  VectorParamsAs1DForOutWhenUnconnected=off
  wires:
  In1/1 -> He Selector/1
  Mux/1 -> Out1/1
  Logarithmic Wind model/1(uwind) -> Mux/1  "uwind"
  Logarithmic Wind model/2(vwind) -> Mux/2  "vwind"
  Logarithmic Wind model/3(wwind) -> Mux/3  "wwind"
  He Selector/1 -> Logarithmic Wind model/1(he)

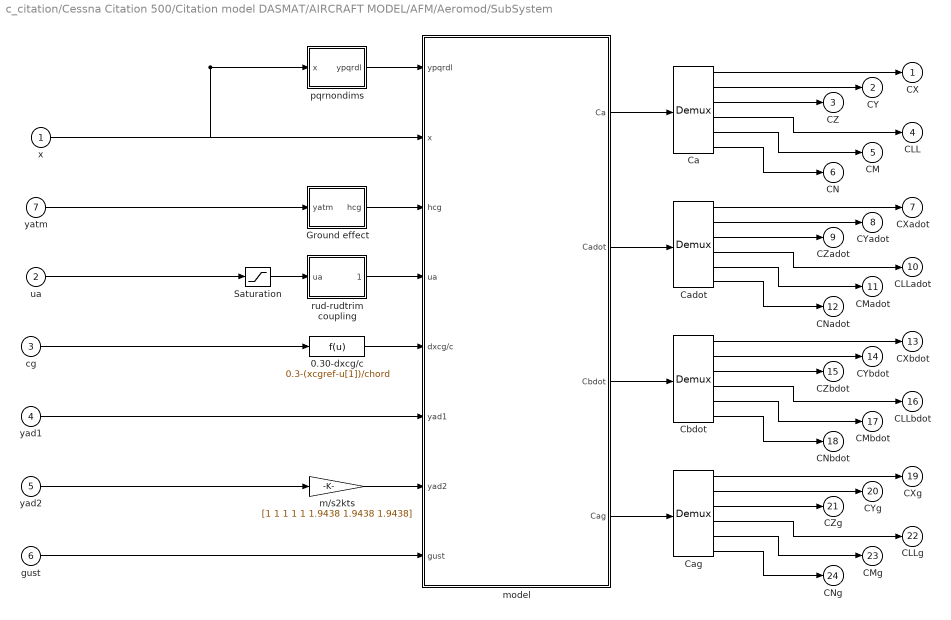
== system c_citation/Cessna Citation 500/Citation model DASMAT/AIRCRAFT MODEL/AFM/Aeromod/SubSystem ==
  x : Inport
  ua : Inport  Port=2
  cg : Inport  Port=3
  yad1 : Inport  Port=4
  yad2 : Inport  Port=5
  gust : Inport  Port=6
  yatm : Inport  Port=7
  0.30-dxcg/c : Fcn  Expr=0.3-(xcgref-u[1])/chord
  Ca : Demux  Outputs=6
      settings: DisplayOption=none
  Cadot : Demux  Outputs=6
      settings: DisplayOption=none
  Cag : Demux  Outputs=6
      settings: DisplayOption=none
  Cbdot : Demux  Outputs=6
      settings: DisplayOption=none
  Ground effect : Subsystem
  Saturation : Saturate  UpperLimit="[ 15  37  22  15  20  10 40 180/pi]*pi/180"  LowerLimit="[-20 -37 -22 -15 -20 -10 0  0]*pi/180"
  m/s2kts : Gain  Gain=[1 1 1 1 1 1.9438 1.9438 1.9438]  SaturateOnIntegerOverflow=on  OutDataTypeStr=Inherit: Same as input  ParamDataTypeStr=Inherit: Same as input
  model : Subsystem
  pqrnondims : Subsystem
  rud-rudtrim coupling : Subsystem
  CX : Outport  VectorParamsAs1DForOutWhenUnconnected=off
  CY : Outport  Port=2  VectorParamsAs1DForOutWhenUnconnected=off
  CZ : Outport  Port=3  VectorParamsAs1DForOutWhenUnconnected=off
  CLL : Outport  Port=4  VectorParamsAs1DForOutWhenUnconnected=off
  CM : Outport  Port=5  VectorParamsAs1DForOutWhenUnconnected=off
  CN : Outport  Port=6  VectorParamsAs1DForOutWhenUnconnected=off
  CXadot : Outport  Port=7  VectorParamsAs1DForOutWhenUnconnected=off
  CYadot : Outport  Port=8  VectorParamsAs1DForOutWhenUnconnected=off
  CZadot : Outport  Port=9  VectorParamsAs1DForOutWhenUnconnected=off
  CLLadot : Outport  Port=10  VectorParamsAs1DForOutWhenUnconnected=off
  CMadot : Outport  Port=11  VectorParamsAs1DForOutWhenUnconnected=off
  CNadot : Outport  Port=12  VectorParamsAs1DForOutWhenUnconnected=off
  CXbdot : Outport  Port=13  VectorParamsAs1DForOutWhenUnconnected=off
  CYbdot : Outport  Port=14  VectorParamsAs1DForOutWhenUnconnected=off
  CZbdot : Outport  Port=15  VectorParamsAs1DForOutWhenUnconnected=off
  CLLbdot : Outport  Port=16  VectorParamsAs1DForOutWhenUnconnected=off
  CMbdot : Outport  Port=17  VectorParamsAs1DForOutWhenUnconnected=off
  CNbdot : Outport  Port=18  VectorParamsAs1DForOutWhenUnconnected=off
  CXg : Outport  Port=19  VectorParamsAs1DForOutWhenUnconnected=off
  CYg : Outport  Port=20  VectorParamsAs1DForOutWhenUnconnected=off
  CZg : Outport  Port=21  VectorParamsAs1DForOutWhenUnconnected=off
  CLLg : Outport  Port=22  VectorParamsAs1DForOutWhenUnconnected=off
  CMg : Outport  Port=23  VectorParamsAs1DForOutWhenUnconnected=off
  CNg : Outport  Port=24  VectorParamsAs1DForOutWhenUnconnected=off
  wires:
  yad2/1 -> m/s2kts/1
  m/s2kts/1 -> model/7(yad2)
  Saturation/1 -> rud-rudtrim coupling/1(ua)
  model/4(Cag) -> Cag/1
  model/3(Cbdot) -> Cbdot/1
  Cbdot/2 -> CYbdot/1
  Cbdot/1 -> CXbdot/1
  Cbdot/3 -> CZbdot/1
  Cbdot/4 -> CLLbdot/1
  Cbdot/5 -> CMbdot/1
  Cbdot/6 -> CNbdot/1
  Cag/6 -> CNg/1
  Cag/5 -> CMg/1
  Cag/4 -> CLLg/1
  Cag/3 -> CZg/1
  Cag/1 -> CXg/1
  Cag/2 -> CYg/1
  model/2(Cadot) -> Cadot/1
  Cadot/2 -> CYadot/1
  Cadot/1 -> CXadot/1
  Cadot/3 -> CZadot/1
  Cadot/4 -> CLLadot/1
  Cadot/5 -> CMadot/1
  Cadot/6 -> CNadot/1
  Ca/6 -> CN/1
  Ca/5 -> CM/1
  Ca/4 -> CLL/1
  Ca/3 -> CZ/1
  Ca/1 -> CX/1
  Ca/2 -> CY/1
  model/1(Ca) -> Ca/1
  yad1/1 -> model/6(yad1)
  gust/1 -> model/8(gust)
  cg/1 -> 0.30-dxcg/c/1
  ua/1 -> Saturation/1
  x/1 -> pqrnondims/1(x), model/2(x)
  0.30-dxcg/c/1 -> model/5(dxcg/c)
  Ground effect/1(hcg) -> model/3(hcg)
  rud-rudtrim coupling/1(ua coupled) -> model/4(ua)
  pqrnondims/1(ypqrdl) -> model/1(ypqrdl)
  yatm/1 -> Ground effect/1(yatm)

== system c_citation/Cessna Citation 500/Citation model DASMAT/AIRCRAFT MODEL/AFM/FMaerodims/dims ==
  note: X,Y,Z
  FM/length : Inport
  Demux : Demux  Outputs=[12 3 3 3 3]
      settings: DisplayOption=none
  LL,M,N air : Gain  Gain=[span chord span]  SaturateOnIntegerOverflow=on  OutDataTypeStr=Inherit: Same as input  ParamDataTypeStr=Inherit: Same as input
  LL,M,N body : Gain  Gain=[span chord span]  SaturateOnIntegerOverflow=on  OutDataTypeStr=Inherit: Same as input  ParamDataTypeStr=Inherit: Same as input
  LL,M,N earth : Gain  Gain=[span chord span]  SaturateOnIntegerOverflow=on  OutDataTypeStr=Inherit: Same as input  ParamDataTypeStr=Inherit: Same as input
  LL,M,N stab : Gain  Gain=[span chord span]  SaturateOnIntegerOverflow=on  OutDataTypeStr=Inherit: Same as input  ParamDataTypeStr=Inherit: Same as input
  Mux : Mux  Inputs=[12 3 3 3 3]
  FM : Outport  VectorParamsAs1DForOutWhenUnconnected=off
  wires:
  LL,M,N earth/1 -> Mux/5
  Demux/5 -> LL,M,N earth/1
  LL,M,N body/1 -> Mux/4
  LL,M,N stab/1 -> Mux/3
  LL,M,N air/1 -> Mux/2
  Demux/1 -> Mux/1
  Demux/2 -> LL,M,N air/1
  Demux/3 -> LL,M,N stab/1
  Demux/4 -> LL,M,N body/1
  Mux/1 -> FM/1
  FM/length/1 -> Demux/1

== system c_citation/Cessna Citation 500/Citation model DASMAT/AIRCRAFT MODEL/AFM/FMaerodims/dims1 ==
  note: X,Y,Z
  F FM/length : Inport
  Demux : Demux  Outputs=[12 3 3 3 3]
      settings: DisplayOption=none
  LL,M,N air : Gain  Gain=[span chord span]  SaturateOnIntegerOverflow=on  OutDataTypeStr=Inherit: Same as input  ParamDataTypeStr=Inherit: Same as input
  LL,M,N body : Gain  Gain=[span chord span]  SaturateOnIntegerOverflow=on  OutDataTypeStr=Inherit: Same as input  ParamDataTypeStr=Inherit: Same as input
  LL,M,N earth : Gain  Gain=[span chord span]  SaturateOnIntegerOverflow=on  OutDataTypeStr=Inherit: Same as input  ParamDataTypeStr=Inherit: Same as input
  LL,M,N stab : Gain  Gain=[span chord span]  SaturateOnIntegerOverflow=on  OutDataTypeStr=Inherit: Same as input  ParamDataTypeStr=Inherit: Same as input
  Mux : Mux  Inputs=[12 3 3 3 3]
  FM : Outport  VectorParamsAs1DForOutWhenUnconnected=off
  wires:
  F FM/length/1 -> Demux/1
  Mux/1 -> FM/1
  Demux/4 -> LL,M,N body/1
  Demux/3 -> LL,M,N stab/1
  Demux/2 -> LL,M,N air/1
  Demux/1 -> Mux/1
  LL,M,N air/1 -> Mux/2
  LL,M,N stab/1 -> Mux/3
  LL,M,N body/1 -> Mux/4
  Demux/5 -> LL,M,N earth/1
  LL,M,N earth/1 -> Mux/5

== system c_citation/Cessna Citation 500/Citation model DASMAT/AIRCRAFT MODEL/AFM/FMaerodims/dims2 ==
  note: X,Y,Z
  F FM/length : Inport
  Demux : Demux  Outputs=[12 3 3 3 3]
      settings: DisplayOption=none
  LL,M,N air : Gain  Gain=[span chord span]  SaturateOnIntegerOverflow=on  OutDataTypeStr=Inherit: Same as input  ParamDataTypeStr=Inherit: Same as input
  LL,M,N body : Gain  Gain=[span chord span]  SaturateOnIntegerOverflow=on  OutDataTypeStr=Inherit: Same as input  ParamDataTypeStr=Inherit: Same as input
  LL,M,N earth : Gain  Gain=[span chord span]  SaturateOnIntegerOverflow=on  OutDataTypeStr=Inherit: Same as input  ParamDataTypeStr=Inherit: Same as input
  LL,M,N stab : Gain  Gain=[span chord span]  SaturateOnIntegerOverflow=on  OutDataTypeStr=Inherit: Same as input  ParamDataTypeStr=Inherit: Same as input
  Mux : Mux  Inputs=[12 3 3 3 3]
  FM : Outport  VectorParamsAs1DForOutWhenUnconnected=off
  wires:
  LL,M,N earth/1 -> Mux/5
  Demux/5 -> LL,M,N earth/1
  LL,M,N body/1 -> Mux/4
  LL,M,N stab/1 -> Mux/3
  LL,M,N air/1 -> Mux/2
  Demux/1 -> Mux/1
  Demux/2 -> LL,M,N air/1
  Demux/3 -> LL,M,N stab/1
  Demux/4 -> LL,M,N body/1
  Mux/1 -> FM/1
  F FM/length/1 -> Demux/1

== system c_citation/Cessna Citation 500/Citation model DASMAT/AIRCRAFT MODEL/AFM/FMgustdims/dims ==
  note: X,Y,Z
  F M/length : Inport
  Demux : Demux  Outputs=[12 3 3 3 3]
      settings: DisplayOption=none
  LL,M,N air : Gain  Gain=[span chord span]  SaturateOnIntegerOverflow=on  OutDataTypeStr=Inherit: Same as input  ParamDataTypeStr=Inherit: Same as input
  LL,M,N body : Gain  Gain=[span chord span]  SaturateOnIntegerOverflow=on  OutDataTypeStr=Inherit: Same as input  ParamDataTypeStr=Inherit: Same as input
  LL,M,N earth : Gain  Gain=[span chord span]  SaturateOnIntegerOverflow=on  OutDataTypeStr=Inherit: Same as input  ParamDataTypeStr=Inherit: Same as input
  LL,M,N stab : Gain  Gain=[span chord span]  SaturateOnIntegerOverflow=on  OutDataTypeStr=Inherit: Same as input  ParamDataTypeStr=Inherit: Same as input
  Mux : Mux  Inputs=[12 3 3 3 3]
  FM : Outport  VectorParamsAs1DForOutWhenUnconnected=off
  wires:
  LL,M,N earth/1 -> Mux/5
  Demux/5 -> LL,M,N earth/1
  LL,M,N body/1 -> Mux/4
  LL,M,N stab/1 -> Mux/3
  LL,M,N air/1 -> Mux/2
  Demux/1 -> Mux/1
  Demux/2 -> LL,M,N air/1
  Demux/3 -> LL,M,N stab/1
  Demux/4 -> LL,M,N body/1
  Mux/1 -> FM/1
  F M/length/1 -> Demux/1

== system c_citation/Cessna Citation 500/Citation model DASMAT/AIRCRAFT MODEL/EFM/Engmod/Citation eng_mod ==
  In1 : Inport
  Demux : Demux  Outputs=32
      settings: DisplayOption=none
  Mux : Mux  Inputs=6
  Mux1 : Mux  Inputs=2
  Subsystem1 : Subsystem
  Out1 : Outport  VectorParamsAs1DForOutWhenUnconnected=off
  ypp : Outport  Port=2  VectorParamsAs1DForOutWhenUnconnected=off
  wires:
  Subsystem1/4(MXt) -> Mux/4
  Subsystem1/3(Zt) -> Mux/3
  Subsystem1/2(Yt) -> Mux/2
  Subsystem1/1(Xt) -> Mux/1
  Subsystem1/6(MZt) -> Mux/6
  Subsystem1/5(MYt) -> Mux/5
  Mux/1 -> Out1/1
  In1/1 -> Demux/1
  Demux/1 -> Subsystem1/1(pbody)
  Demux/2 -> Subsystem1/2(qbody)
  Demux/3 -> Subsystem1/3(rbody)
  Demux/4 -> Subsystem1/4(VTAS)
  Demux/5 -> Subsystem1/5(alpha)
  Demux/6 -> Subsystem1/6(beta)
  Demux/7 -> Subsystem1/7(phi)
  Demux/8 -> Subsystem1/8(theta)
  Demux/9 -> Subsystem1/9(psi)
  Demux/10 -> Subsystem1/10(he)
  Demux/11 -> Subsystem1/11(xe)
  Demux/12 -> Subsystem1/12(ye)
  Demux/13 -> Subsystem1/13(ut1)
  Demux/14 -> Subsystem1/14(ut2)
  Demux/15 -> Subsystem1/15(pstat)
  Demux/16 -> Subsystem1/16(rho)
  Demux/17 -> Subsystem1/17(temp)
  Demux/18 -> Subsystem1/18(grav)
  Demux/19 -> Subsystem1/19(hpress)
  Demux/20 -> Subsystem1/20(hradio)
  Demux/21 -> Subsystem1/21(Hgeopot)
  Demux/22 -> Subsystem1/22(Vsound)
  Demux/23 -> Subsystem1/23(Mach)
  Demux/24 -> Subsystem1/24(qdyn)
  Demux/25 -> Subsystem1/25(Reynl)
  Demux/26 -> Subsystem1/26(qc)
  Demux/27 -> Subsystem1/27(qrel)
  Demux/28 -> Subsystem1/28(ptot)
  Demux/29 -> Subsystem1/29(temptot)
  Demux/30 -> Subsystem1/30(VEAS)
  Demux/31 -> Subsystem1/31(VCAS)
  Demux/32 -> Subsystem1/32(VIAS)
  Subsystem1/7(yppleft) -> Mux1/1
  Subsystem1/8(yppright) -> Mux1/2
  Mux1/1 -> ypp/1

== system c_citation/Cessna Citation 500/Citation model DASMAT/AIRCRAFT MODEL/EQM/State Derivatives/Vabdot ==
  x : Inport
  ypqr : Inport  Port=2
  Ftot : Inport  Port=3
  Fadot : Inport  Port=4
  Fbdot : Inport  Port=5
  mass : Inport  Port=6
  wind : Inport  Port=7
  Mux1 : Mux  Inputs=3
  Prod : Product  InputSameDT=on  SaturateOnIntegerOverflow=on  OutDataTypeStr=Inherit: Same as first input
  Prod1 : Product  InputSameDT=on  SaturateOnIntegerOverflow=on  OutDataTypeStr=Inherit: Same as first input
  Sum : Sum  Inputs=+++  InputSameDT=on  SaturateOnIntegerOverflow=on  OutDataTypeStr=Inherit: Same as first input
  Vdot : Subsystem
  abdot : Subsystem
  winddot : Derivative
  Vabdot : Outport  VectorParamsAs1DForOutWhenUnconnected=off
  Ftot corrected : Outport  Port=2  VectorParamsAs1DForOutWhenUnconnected=off
  wires:
  wind/1 -> winddot/1, Vdot/5(wind), abdot/7(wind)
  winddot/1 -> abdot/8(winddot), Vdot/6(winddot)
  Vdot/1(Vdot) -> Mux1/1
  mass/1 -> Vdot/4(mass), abdot/6(mass)
  ypqr/1 -> Vdot/2(ypqr), abdot/2(ypqr)
  x/1 -> Vdot/1(x), abdot/1(x)
  abdot/1(adot) -> Vdot/7(adot), Prod/2, Mux1/2
  abdot/2(bdot) -> Vdot/8(bdot), Prod1/2, Mux1/3
  Fbdot/1 -> abdot/5(Fbdot), Prod1/1
  Fadot/1 -> abdot/4(Fadot), Prod/1
  Prod1/1 -> Sum/3
  Mux1/1 -> Vabdot/1
  Sum/1 -> Vdot/3(Ftot), Ftot corrected/1
  Prod/1 -> Sum/2
  Ftot/1 -> abdot/3(Ftot), Sum/1

== system c_citation/Cessna Citation 500/Citation model DASMAT/AIRCRAFT MODEL/EQM/State Derivatives/eulerdot ==
  x : Inport
  Mux : Mux  Inputs=3
  phidot : Fcn  Expr=u[1]+tan(u[8])*(u[2]*sin(u[7])+u[3]*cos(u[7]))
  psidot : Fcn  Expr=(u[2]*sin(u[7])+u[3]*cos(u[7]))/cos(u[8])
  thetadot : Fcn  Expr=u[2]*cos(u[7])-u[3]*sin(u[7])
  eulerdot : Outport  VectorParamsAs1DForOutWhenUnconnected=off
  wires:
  x/1 -> phidot/1, psidot/1, thetadot/1
  Mux/1 -> eulerdot/1
  phidot/1 -> Mux/1
  thetadot/1 -> Mux/2
  psidot/1 -> Mux/3

== system c_citation/Cessna Citation 500/Citation model DASMAT/AIRCRAFT MODEL/EQM/State Derivatives/hxydot ==
  yuvw : Inport
  wind : Inport  Port=2
  Demux : Demux  Outputs=[3 3 3 3]
      settings: DisplayOption=none
  Demux1 : Demux  Outputs=[3 3 3 3]
      settings: DisplayOption=none
  Mux : Mux  Inputs=[3 3]
  Mux1 : Mux  Inputs=3
  Terminator_{1..6} (6 alike) : Terminator
  hedot : Fcn  Expr=-(u[3]+u[6])
  xedot : Fcn  Expr=u[1]+u[4]
  yedot : Fcn  Expr=u[2]+u[5]
  hxydot : Outport  VectorParamsAs1DForOutWhenUnconnected=off
  wires:
  Demux1/3 -> Terminator_6/1
  Demux1/2 -> Terminator_5/1
  Demux1/1 -> Terminator_4/1
  Demux/3 -> Terminator_3/1
  Demux/2 -> Terminator_2/1
  Demux/1 -> Terminator_1/1
  wind/1 -> Demux1/1
  Demux1/4 -> Mux/2
  yedot/1 -> Mux1/3
  xedot/1 -> Mux1/2
  hedot/1 -> Mux1/1  "hedot"
  Mux1/1 -> hxydot/1
  Mux/1 -> hedot/1, yedot/1, xedot/1
  yuvw/1 -> Demux/1
  Demux/4 -> Mux/1

== system c_citation/Cessna Citation 500/Citation model DASMAT/AIRCRAFT MODEL/EQM/State Derivatives/mass properties ==
  massinit : Inport
  GAMMA : Fcn  Expr=u[1]*u[3]-u[4]*u[4]
  Mux : Mux  Inputs=[4 1]
  Mux1 : Mux  Inputs=9
  Terminator_1 : Terminator
  c1 : Fcn  Expr=((u[2]-u[3])*u[3]-u[4]*u[4])/u[5]
  c2 : Fcn  Expr=(u[1]-u[2]+u[3])*u[4]/u[5]
  c3 : Fcn  Expr=u[3]/u[5]
  c4 : Fcn  Expr=u[4]/u[5]
  c5 : Fcn  Expr=(u[3]-u[1])/u[2]
  c6 : Fcn  Expr=u[4]/u[2]
  c7 : Fcn  Expr=1/u[2]
  c8 : Fcn  Expr=((u[1]-u[2])*u[1]+u[4]*u[4])/u[5]
  c9 : Fcn  Expr=u[1]/u[5]
  mass cg inertia : Demux  Outputs=[1 3 4]
      settings: DisplayOption=none
  mass : Outport  VectorParamsAs1DForOutWhenUnconnected=off
  inertia : Outport  Port=2  VectorParamsAs1DForOutWhenUnconnected=off
  wires:
  mass cg inertia/2 -> Terminator_1/1
  massinit/1 -> mass cg inertia/1
  mass cg inertia/1 -> mass/1
  mass cg inertia/3 -> GAMMA/1, Mux/1
  GAMMA/1 -> Mux/2
  c1/1 -> Mux1/1
  c2/1 -> Mux1/2
  c3/1 -> Mux1/3
  c4/1 -> Mux1/4
  c5/1 -> Mux1/5
  c6/1 -> Mux1/6
  c7/1 -> Mux1/7
  c8/1 -> Mux1/8
  c9/1 -> Mux1/9
  Mux1/1 -> inertia/1
  Mux/1 -> c2/1, c3/1, c4/1, c5/1, c6/1, c7/1, c8/1, c9/1, c1/1

== system c_citation/Cessna Citation 500/Citation model DASMAT/AIRCRAFT MODEL/EQM/State Derivatives/pqrdot ==
  ypqr : Inport
  Mtot : Inport  Port=2
  Madot : Inport  Port=3
  Mbdot : Inport  Port=4
  inertia : Inport  Port=5
  Vabdot : Inport  Port=6
  Demux : Demux  Outputs=3
      settings: DisplayOption=none
  Demux1 : Demux  Outputs=[3 3 3 3]
      settings: DisplayOption=none
  Demux2 : Demux  Outputs=[3 3 3 3]
      settings: DisplayOption=none
  Mux : Mux  Inputs=[3 3 9]
  Mux1 : Mux  Inputs=3
  Prod : Product  InputSameDT=on  SaturateOnIntegerOverflow=on  OutDataTypeStr=Inherit: Same as first input
  Prod1 : Product  InputSameDT=on  SaturateOnIntegerOverflow=on  OutDataTypeStr=Inherit: Same as first input
  Sum : Sum  Inputs=+++  InputSameDT=on  SaturateOnIntegerOverflow=on  OutDataTypeStr=Inherit: Same as first input
  Terminator_{1..7} (7 alike) : Terminator
  pdot : Fcn  Expr=(u[7]*u[3]+u[8]*u[1])*u[2]+u[9]*u[4]+u[10]*u[6]
  qdot : Fcn  Expr=u[11]*u[1]*u[3]-u[12]*(u[1]^2-u[3]^2)+u[13]*u[5]
  rdot : Fcn  Expr=(u[14]*u[1]-u[8]*u[3])*u[2]+u[10]*u[4]+u[15]*u[6]
  pqrdot : Outport  VectorParamsAs1DForOutWhenUnconnected=off
  Mtot corrected : Outport  Port=2  VectorParamsAs1DForOutWhenUnconnected=off
  wires:
  Demux2/4 -> Terminator_7/1
  Demux2/2 -> Terminator_6/1
  Demux2/1 -> Terminator_5/1
  Demux1/4 -> Terminator_4/1
  Demux1/2 -> Terminator_3/1
  Demux1/1 -> Terminator_2/1
  Demux/1 -> Terminator_1/1
  Demux2/3 -> Mux/2
  Demux1/3 -> Mux/1
  inertia/1 -> Mux/3
  qdot/1 -> Mux1/2
  pdot/1 -> Mux1/1
  Mux/1 -> pdot/1, rdot/1, qdot/1
  Mux1/1 -> pqrdot/1
  ypqr/1 -> Demux1/1
  Demux/3 -> Prod1/2
  Demux/2 -> Prod/2
  Mbdot/1 -> Prod1/1
  Madot/1 -> Prod/1
  Mtot/1 -> Sum/1
  Vabdot/1 -> Demux/1
  Prod1/1 -> Sum/3
  Sum/1 -> Demux2/1, Mtot corrected/1
  Prod/1 -> Sum/2
  rdot/1 -> Mux1/3

== system c_citation/Cessna Citation 500/Citation model DASMAT/AIRCRAFT MODEL/EQM/State Derivatives/states transformation ==
  x : Inport
  1/V : Fcn  Expr=1/u[4]
  Demux : Demux  Outputs=[3 3 3 3]
      settings: DisplayOption=none
  Mux : Mux  Inputs=[12 1 1 1]
  Mux1 : Mux  Inputs=[12 1 1 1]
  Mux2 : Mux  Inputs=3
  Mux3 : Mux  Inputs=[3 3 3 3 12]
  Prod{,1..4} (5 alike) : Product  InputSameDT=on  SaturateOnIntegerOverflow=on  OutDataTypeStr=Inherit: Same as first input
  Terminator_{1..8} (8 alike) : Terminator
  Vab transformation : S-Function  FunctionName=ac_axes  Parameters=0  SFunctionDeploymentMode=off  EnableBusSupport=off
  b/2V : Fcn  Expr=span/(2*u[4])
  b/2V1 : Fcn  Expr=span/(2*u[4])
  c/V : Fcn  Expr=chord/u[4]
  pqr transformation : S-Function  FunctionName=ac_axes  Parameters=2  SFunctionDeploymentMode=off  EnableBusSupport=off
  states : Demux  Outputs=12
      settings: DisplayOption=none
  zero : Constant  Value=0
  ypqr : Outport  VectorParamsAs1DForOutWhenUnconnected=off
  yuvw : Outport  Port=2  VectorParamsAs1DForOutWhenUnconnected=off
  ydl : Outport  Port=3  VectorParamsAs1DForOutWhenUnconnected=off
  wires:
  states/12 -> Terminator_8/1
  states/11 -> Terminator_7/1
  states/10 -> Terminator_6/1
  states/9 -> Terminator_5/1
  states/8 -> Terminator_4/1
  states/7 -> Terminator_3/1
  states/6 -> Terminator_2/1
  states/5 -> Terminator_1/1
  states/3 -> Mux/4
  states/2 -> Mux/3
  states/1 -> Mux/2
  Mux/1 -> pqr transformation/1
  Mux1/1 -> Vab transformation/1
  zero/1 -> Mux1/3, Mux1/4
  states/4 -> Mux1/2
  c/V/1 -> Mux2/2
  b/2V1/1 -> Mux2/3
  b/2V/1 -> Mux2/1
  Demux/1 -> Prod/1
  Demux/2 -> Prod1/1
  Demux/3 -> Prod2/1
  Demux/4 -> Prod3/1
  1/V/1 -> Prod4/2
  pqr transformation/1 -> Demux/1, ypqr/1
  Vab transformation/1 -> Prod4/1, yuvw/1
  Mux2/1 -> Prod1/2, Prod/2, Prod2/2, Prod3/2
  Prod/1 -> Mux3/1
  Prod1/1 -> Mux3/2
  Prod2/1 -> Mux3/3
  Prod3/1 -> Mux3/4
  Prod4/1 -> Mux3/5
  Mux3/1 -> ydl/1
  x/1 -> Mux/1, Mux1/1, b/2V/1, b/2V1/1, c/V/1, 1/V/1, states/1

== system c_citation/Cessna Citation 500/Citation model DASMAT/AIRCRAFT MODEL/LANDING GEAR/Landing Gear model/Correct for terrain elevation ==
  x : Inport
  terr elev : Inport  Port=2
  Demux : Demux  Outputs=[9 1 2]
      settings: DisplayOption=none
  Mux : Mux  Inputs=3
  terrain elevation corr : Sum  Inputs=-+|  SaturateOnIntegerOverflow=on
  x corrected : Outport  VectorParamsAs1DForOutWhenUnconnected=off
  wires:
  x/1 -> Demux/1
  Demux/1 -> Mux/1
  Demux/3 -> Mux/3
  Mux/1 -> x corrected/1
  Demux/2 -> terrain elevation corr/2
  terr elev/1 -> terrain elevation corr/1
  terrain elevation corr/1 -> Mux/2
